simulink model "TST_WESDem_CalcState"  (R2016b)
settings: Solver=FixedStepDiscrete  StartTime=0.0  StopTime=simTime  FixedStep=sampleTime  RelTol=1e-3
values from neighbouring files (symbols this model uses):
  testCase = 1    [initTST_WESDem_CalcState_001.m]    (also in initTST_WESDem_CalcState_002.m = 2; initTST_WESDem_CalcState_003.m = 3)
libraries: simulink x25, UnitTest_Lib x21
(part 1 of 2)
settings Model: Creator=zhengjinyan  LastModifiedBy=zhengjinyan
settings DebuggingCC: SignalRangeChecking=error

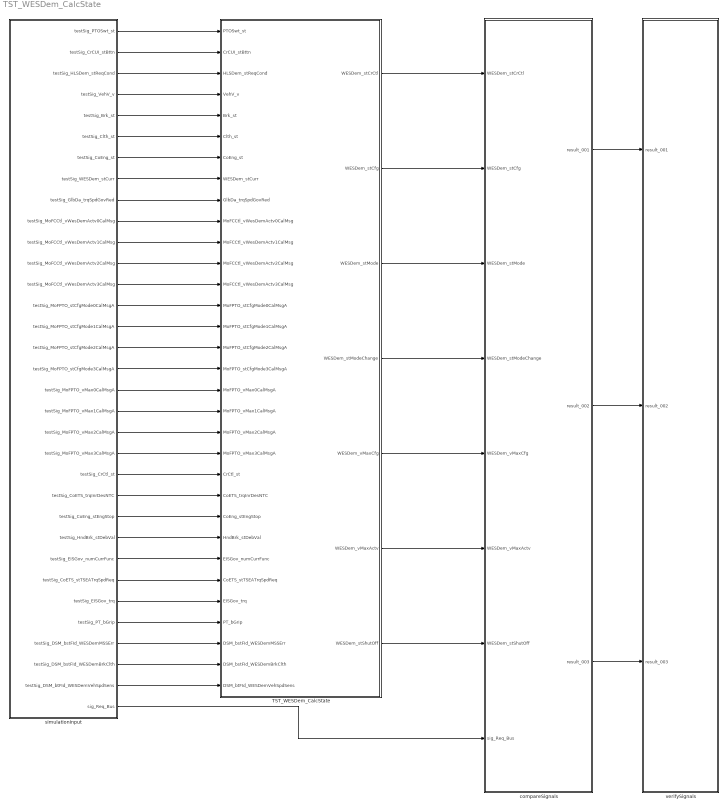
== system TST_WESDem_CalcState ==
  TST_WESDem_CalcState : Subsystem
  compareSignals : Subsystem
  simulationInput : Subsystem
  verifySignals : Subsystem
  wires:
  simulationInput/1(testSig_PTOSwt_st) -> TST_WESDem_CalcState/1(PTOSwt_st)
  simulationInput/2(testSig_CrCUI_stBttn) -> TST_WESDem_CalcState/2(CrCUI_stBttn)
  simulationInput/3(testSig_HLSDem_stReqCond) -> TST_WESDem_CalcState/3(HLSDem_stReqCond)
  simulationInput/4(testSig_VehV_v) -> TST_WESDem_CalcState/4(VehV_v)
  simulationInput/5(testSig_Brk_st) -> TST_WESDem_CalcState/5(Brk_st)
  simulationInput/6(testSig_Clth_st) -> TST_WESDem_CalcState/6(Clth_st)
  simulationInput/7(testSig_CoEng_st) -> TST_WESDem_CalcState/7(CoEng_st)
  simulationInput/8(testSig_WESDem_stCurr) -> TST_WESDem_CalcState/8(WESDem_stCurr)
  simulationInput/9(testSig_GlbDa_trqSpdGovRed) -> TST_WESDem_CalcState/9(GlbDa_trqSpdGovRed)
  simulationInput/10(testSig_MoFCCtl_vWesDemActv0CalMsg) -> TST_WESDem_CalcState/10(MoFCCtl_vWesDemActv0CalMsg)
  simulationInput/11(testSig_MoFCCtl_vWesDemActv1CalMsg) -> TST_WESDem_CalcState/11(MoFCCtl_vWesDemActv1CalMsg)
  simulationInput/12(testSig_MoFCCtl_vWesDemActv2CalMsg) -> TST_WESDem_CalcState/12(MoFCCtl_vWesDemActv2CalMsg)
  simulationInput/13(testSig_MoFCCtl_vWesDemActv3CalMsg) -> TST_WESDem_CalcState/13(MoFCCtl_vWesDemActv3CalMsg)
  simulationInput/14(testSig_MoFPTO_stCfgMode0CalMsgA) -> TST_WESDem_CalcState/14(MoFPTO_stCfgMode0CalMsgA)
  simulationInput/15(testSig_MoFPTO_stCfgMode1CalMsgA) -> TST_WESDem_CalcState/15(MoFPTO_stCfgMode1CalMsgA)
  simulationInput/16(testSig_MoFPTO_stCfgMode2CalMsgA) -> TST_WESDem_CalcState/16(MoFPTO_stCfgMode2CalMsgA)
  simulationInput/17(testSig_MoFPTO_stCfgMode3CalMsgA) -> TST_WESDem_CalcState/17(MoFPTO_stCfgMode3CalMsgA)
  simulationInput/18(testSig_MoFPTO_vMax0CalMsgA) -> TST_WESDem_CalcState/18(MoFPTO_vMax0CalMsgA)
  simulationInput/19(testSig_MoFPTO_vMax1CalMsgA) -> TST_WESDem_CalcState/19(MoFPTO_vMax1CalMsgA)
  simulationInput/20(testSig_MoFPTO_vMax2CalMsgA) -> TST_WESDem_CalcState/20(MoFPTO_vMax2CalMsgA)
  simulationInput/21(testSig_MoFPTO_vMax3CalMsgA) -> TST_WESDem_CalcState/21(MoFPTO_vMax3CalMsgA)
  simulationInput/22(testSig_CrCtl_st) -> TST_WESDem_CalcState/22(CrCtl_st)
  simulationInput/23(testSig_CoETS_trqInrDesNTC) -> TST_WESDem_CalcState/23(CoETS_trqInrDesNTC)
  simulationInput/24(testSig_CoEng_stEngStop) -> TST_WESDem_CalcState/24(CoEng_stEngStop)
  simulationInput/25(testSig_HndBrk_stDebVal) -> TST_WESDem_CalcState/25(HndBrk_stDebVal)
  simulationInput/26(testSig_EISGov_numCurrFunc) -> TST_WESDem_CalcState/26(EISGov_numCurrFunc)
  simulationInput/27(testSig_CoETS_stTSEATrqSpdReq) -> TST_WESDem_CalcState/27(CoETS_stTSEATrqSpdReq)
  simulationInput/28(testSig_EISGov_trq) -> TST_WESDem_CalcState/28(EISGov_trq)
  simulationInput/29(testSig_PT_bGrip) -> TST_WESDem_CalcState/29(PT_bGrip)
  simulationInput/30(testSig_DSM_bstFId_WESDemMSSErr) -> TST_WESDem_CalcState/30(DSM_bstFId_WESDemMSSErr)
  simulationInput/31(testSig_DSM_bstFId_WESDemBrkClth) -> TST_WESDem_CalcState/31(DSM_bstFId_WESDemBrkClth)
  simulationInput/32(testSig_DSM_btFId_WESDemVehSpdSens) -> TST_WESDem_CalcState/32(DSM_btFId_WESDemVehSpdSens)
  TST_WESDem_CalcState/1(WESDem_stCrCtl) -> compareSignals/1(WESDem_stCrCtl)
  TST_WESDem_CalcState/2(WESDem_stCfg) -> compareSignals/2(WESDem_stCfg)
  TST_WESDem_CalcState/3(WESDem_stMode) -> compareSignals/3(WESDem_stMode)
  TST_WESDem_CalcState/4(WESDem_stModeChange) -> compareSignals/4(WESDem_stModeChange)
  TST_WESDem_CalcState/5(WESDem_vMaxCfg) -> compareSignals/5(WESDem_vMaxCfg)
  TST_WESDem_CalcState/6(WESDem_vMaxActv) -> compareSignals/6(WESDem_vMaxActv)
  TST_WESDem_CalcState/7(WESDem_stShutOff) -> compareSignals/7(WESDem_stShutOff)
  simulationInput/33(sig_Req_Bus) -> compareSignals/8(sig_Req_Bus)
  compareSignals/1(result_001) -> verifySignals/1(result_001)
  compareSignals/2(result_002) -> verifySignals/2(result_002)
  compareSignals/3(result_003) -> verifySignals/3(result_003)

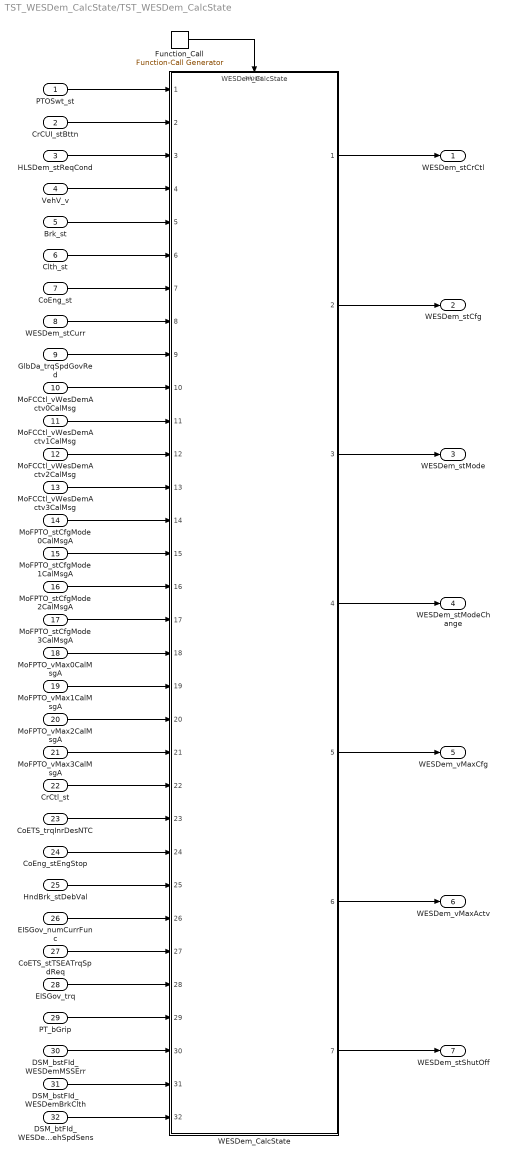
== system TST_WESDem_CalcState/TST_WESDem_CalcState ==
  PTOSwt_st : Inport
  CrCUI_stBttn : Inport  Port=2
  HLSDem_stReqCond : Inport  Port=3
  VehV_v : Inport  Port=4
  Brk_st : Inport  Port=5
  Clth_st : Inport  Port=6
  CoEng_st : Inport  Port=7
  WESDem_stCurr : Inport  Port=8
  GlbDa_trqSpdGovRed : Inport  Port=9
  MoFCCtl_vWesDemActv0CalMsg : Inport  Port=10
  MoFCCtl_vWesDemActv1CalMsg : Inport  Port=11
  MoFCCtl_vWesDemActv2CalMsg : Inport  Port=12
  MoFCCtl_vWesDemActv3CalMsg : Inport  Port=13
  MoFPTO_stCfgMode0CalMsgA : Inport  Port=14
  MoFPTO_stCfgMode1CalMsgA : Inport  Port=15
  MoFPTO_stCfgMode2CalMsgA : Inport  Port=16
  MoFPTO_stCfgMode3CalMsgA : Inport  Port=17
  MoFPTO_vMax0CalMsgA : Inport  Port=18
  MoFPTO_vMax1CalMsgA : Inport  Port=19
  MoFPTO_vMax2CalMsgA : Inport  Port=20
  MoFPTO_vMax3CalMsgA : Inport  Port=21
  CrCtl_st : Inport  Port=22
  CoETS_trqInrDesNTC : Inport  Port=23
  CoEng_stEngStop : Inport  Port=24
  HndBrk_stDebVal : Inport  Port=25
  EISGov_numCurrFunc : Inport  Port=26
  CoETS_stTSEATrqSpdReq : Inport  Port=27
  EISGov_trq : Inport  Port=28
  PT_bGrip : Inport  Port=29
  DSM_bstFId_WESDemMSSErr : Inport  Port=30
  DSM_bstFId_WESDemBrkClth : Inport  Port=31
  DSM_btFId_WESDemVehSpdSens : Inport  Port=32
  Function_Call : simulink/Ports & Subsystems/Function-Call Generator  sample_time=sampleTime  numberOfIterations=1
  WESDem_CalcState : ModelReference  ModelNameDialog=WESDem_CalcState  SimulationMode=Normal  ModelReferenceVersion=1.157  TriggerPortName=function  TriggerPortTriggerType=function-call  TriggerPortStatesWhenEnabling=held
  WESDem_stCrCtl : Outport
  WESDem_stCfg : Outport  Port=2
  WESDem_stMode : Outport  Port=3
  WESDem_stModeChange : Outport  Port=4
  WESDem_vMaxCfg : Outport  Port=5
  WESDem_vMaxActv : Outport  Port=6
  WESDem_stShutOff : Outport  Port=7
  wires:
  Function_Call/1 -> WESDem_CalcState/Trigger
  PTOSwt_st/1 -> WESDem_CalcState/1
  CrCUI_stBttn/1 -> WESDem_CalcState/2
  HLSDem_stReqCond/1 -> WESDem_CalcState/3
  VehV_v/1 -> WESDem_CalcState/4
  Brk_st/1 -> WESDem_CalcState/5
  Clth_st/1 -> WESDem_CalcState/6
  CoEng_st/1 -> WESDem_CalcState/7
  WESDem_stCurr/1 -> WESDem_CalcState/8
  GlbDa_trqSpdGovRed/1 -> WESDem_CalcState/9
  MoFCCtl_vWesDemActv0CalMsg/1 -> WESDem_CalcState/10
  MoFCCtl_vWesDemActv1CalMsg/1 -> WESDem_CalcState/11
  MoFCCtl_vWesDemActv2CalMsg/1 -> WESDem_CalcState/12
  MoFCCtl_vWesDemActv3CalMsg/1 -> WESDem_CalcState/13
  MoFPTO_stCfgMode0CalMsgA/1 -> WESDem_CalcState/14
  MoFPTO_stCfgMode1CalMsgA/1 -> WESDem_CalcState/15
  MoFPTO_stCfgMode2CalMsgA/1 -> WESDem_CalcState/16
  MoFPTO_stCfgMode3CalMsgA/1 -> WESDem_CalcState/17
  MoFPTO_vMax0CalMsgA/1 -> WESDem_CalcState/18
  MoFPTO_vMax1CalMsgA/1 -> WESDem_CalcState/19
  MoFPTO_vMax2CalMsgA/1 -> WESDem_CalcState/20
  MoFPTO_vMax3CalMsgA/1 -> WESDem_CalcState/21
  CrCtl_st/1 -> WESDem_CalcState/22
  CoETS_trqInrDesNTC/1 -> WESDem_CalcState/23
  CoEng_stEngStop/1 -> WESDem_CalcState/24
  HndBrk_stDebVal/1 -> WESDem_CalcState/25
  EISGov_numCurrFunc/1 -> WESDem_CalcState/26
  CoETS_stTSEATrqSpdReq/1 -> WESDem_CalcState/27
  EISGov_trq/1 -> WESDem_CalcState/28
  PT_bGrip/1 -> WESDem_CalcState/29
  DSM_bstFId_WESDemMSSErr/1 -> WESDem_CalcState/30
  DSM_bstFId_WESDemBrkClth/1 -> WESDem_CalcState/31
  DSM_btFId_WESDemVehSpdSens/1 -> WESDem_CalcState/32
  WESDem_CalcState/1 -> WESDem_stCrCtl/1
  WESDem_CalcState/2 -> WESDem_stCfg/1
  WESDem_CalcState/3 -> WESDem_stMode/1
  WESDem_CalcState/4 -> WESDem_stModeChange/1
  WESDem_CalcState/5 -> WESDem_vMaxCfg/1
  WESDem_CalcState/6 -> WESDem_vMaxActv/1
  WESDem_CalcState/7 -> WESDem_stShutOff/1

== system TST_WESDem_CalcState/compareSignals ==
  WESDem_stCrCtl : Inport
  WESDem_stCfg : Inport  Port=2
  WESDem_stMode : Inport  Port=3
  WESDem_stModeChange : Inport  Port=4
  WESDem_vMaxCfg : Inport  Port=5
  WESDem_vMaxActv : Inport  Port=6
  WESDem_stShutOff : Inport  Port=7
  sig_Req_Bus : Inport  Port=8
  BC : BusCreator  Inputs=7
  CTC_001 : simulink/Logic and Bit Operations/Compare To Constant  relop===  const=1  OutDataTypeStr=boolean
  CTC_002 : simulink/Logic and Bit Operations/Compare To Constant  relop===  const=2  OutDataTypeStr=boolean
  CTC_003 : simulink/Logic and Bit Operations/Compare To Constant  relop===  const=3  OutDataTypeStr=boolean
  Requirement_001 : Subsystem
  Requirement_002 : Subsystem
  Requirement_003 : Subsystem
  TC_001 : Constant  Value=testCase
  TC_002 : Constant  Value=testCase
  TC_003 : Constant  Value=testCase
  result_001 : Outport
  result_002 : Outport  Port=2
  result_003 : Outport  Port=3
  wires:
  WESDem_stCrCtl/1 -> BC/1  "WESDem_stCrCtl"
  WESDem_stCfg/1 -> BC/2  "WESDem_stCfg"
  WESDem_stMode/1 -> BC/3  "WESDem_stMode"
  WESDem_stModeChange/1 -> BC/4  "WESDem_stModeChange"
  WESDem_vMaxCfg/1 -> BC/5  "WESDem_vMaxCfg"
  WESDem_vMaxActv/1 -> BC/6  "WESDem_vMaxActv"
  WESDem_stShutOff/1 -> BC/7  "WESDem_stShutOff"
  TC_001/1 -> CTC_001/1
  CTC_001/1 -> Requirement_001/Enable
  sig_Req_Bus/1 -> Requirement_001/2(sig_Req_Bus), Requirement_002/2(sig_Req_Bus), Requirement_003/2(sig_Req_Bus)
  BC/1 -> Requirement_001/1(sig_Result_Bus), Requirement_002/1(sig_Result_Bus), Requirement_003/1(sig_Result_Bus)
  Requirement_001/1(result) -> result_001/1
  TC_002/1 -> CTC_002/1
  CTC_002/1 -> Requirement_002/Enable
  Requirement_002/1(result) -> result_002/1
  TC_003/1 -> CTC_003/1
  CTC_003/1 -> Requirement_003/Enable
  Requirement_003/1(result) -> result_003/1

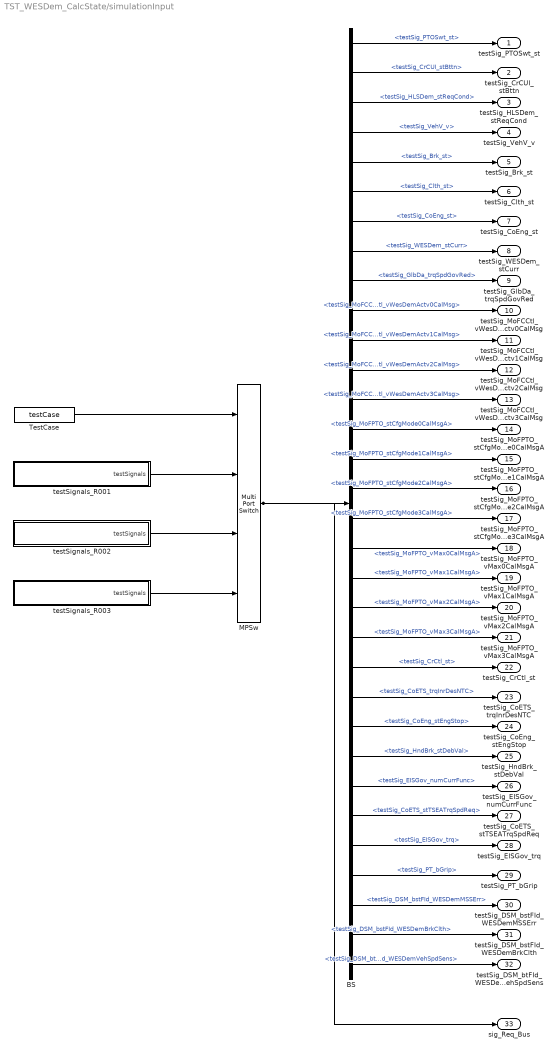
== system TST_WESDem_CalcState/simulationInput ==
  BS : BusSelector  OutputSignals=testSig_PTOSwt_st,testSig_CrCUI_stBttn,testSig_HLSDem_stReqCond,testSig_VehV_v,testSig_Brk_st,testSig_Clth_st,testSig_CoEng_st,testSig_WESDem_stCurr,testSig_GlbDa_trqSpdGovRed,testSig_MoFCCtl_vWesDemActv0CalMsg,testSig_MoFCCtl_vWesDemActv1CalMsg,testSig_MoFCCtl_vWesDemActv2CalMsg,testSig_MoFCCtl_vWesDemActv3CalMsg,testSig_MoFPTO_stCfgMode0CalMsgA,testSig_MoFPTO_stCfgMode1CalMsgA,testSig_MoFPTO_stCfgMode2CalMsgA,testSig_MoFPTO_stCfgMode3CalMsgA,testSig_MoFPTO_vMax0CalMsgA,testSig_MoFPTO_vMax1CalMsgA,testSig_MoFPTO_vMax2CalMsgA,testSig_MoFPTO_vMax3CalMsgA,testSig_CrCtl_st,testSig_CoETS_trqInrDesNTC,testSig_CoEng_stEngStop,testSig_HndBrk_stDebVal,testSig_EISGov_numCurrFunc,testSig_CoETS_stTSEATrqSpdReq,testSig_EISGov_trq,testSig_PT_bGrip,testSig_DSM_bstFId_WESDemMSSErr,testSig_DSM_bstFId_WESDemBrkClth,testSig_DSM_btFId_WESDemVehSpdSens
  MPSw : MultiPortSwitch  SaturateOnIntegerOverflow=on  InputSameDT=on
  TestCase : Constant  Value=testCase
  testSignals_R001 : Subsystem
  testSignals_R002 : Subsystem
  testSignals_R003 : Subsystem
  testSig_PTOSwt_st : Outport
  testSig_CrCUI_stBttn : Outport  Port=2
  testSig_HLSDem_stReqCond : Outport  Port=3
  testSig_VehV_v : Outport  Port=4
  testSig_Brk_st : Outport  Port=5
  testSig_Clth_st : Outport  Port=6
  testSig_CoEng_st : Outport  Port=7
  testSig_WESDem_stCurr : Outport  Port=8
  testSig_GlbDa_trqSpdGovRed : Outport  Port=9
  testSig_MoFCCtl_vWesDemActv0CalMsg : Outport  Port=10
  testSig_MoFCCtl_vWesDemActv1CalMsg : Outport  Port=11
  testSig_MoFCCtl_vWesDemActv2CalMsg : Outport  Port=12
  testSig_MoFCCtl_vWesDemActv3CalMsg : Outport  Port=13
  testSig_MoFPTO_stCfgMode0CalMsgA : Outport  Port=14
  testSig_MoFPTO_stCfgMode1CalMsgA : Outport  Port=15
  testSig_MoFPTO_stCfgMode2CalMsgA : Outport  Port=16
  testSig_MoFPTO_stCfgMode3CalMsgA : Outport  Port=17
  testSig_MoFPTO_vMax0CalMsgA : Outport  Port=18
  testSig_MoFPTO_vMax1CalMsgA : Outport  Port=19
  testSig_MoFPTO_vMax2CalMsgA : Outport  Port=20
  testSig_MoFPTO_vMax3CalMsgA : Outport  Port=21
  testSig_CrCtl_st : Outport  Port=22
  testSig_CoETS_trqInrDesNTC : Outport  Port=23
  testSig_CoEng_stEngStop : Outport  Port=24
  testSig_HndBrk_stDebVal : Outport  Port=25
  testSig_EISGov_numCurrFunc : Outport  Port=26
  testSig_CoETS_stTSEATrqSpdReq : Outport  Port=27
  testSig_EISGov_trq : Outport  Port=28
  testSig_PT_bGrip : Outport  Port=29
  testSig_DSM_bstFId_WESDemMSSErr : Outport  Port=30
  testSig_DSM_bstFId_WESDemBrkClth : Outport  Port=31
  testSig_DSM_btFId_WESDemVehSpdSens : Outport  Port=32
  sig_Req_Bus : Outport  Port=33
  wires:
  BS/1 -> testSig_PTOSwt_st/1  "<testSig_PTOSwt_st>"
  BS/2 -> testSig_CrCUI_stBttn/1  "<testSig_CrCUI_stBttn>"
  BS/3 -> testSig_HLSDem_stReqCond/1  "<testSig_HLSDem_stReqCond>"
  BS/4 -> testSig_VehV_v/1  "<testSig_VehV_v>"
  BS/5 -> testSig_Brk_st/1  "<testSig_Brk_st>"
  BS/6 -> testSig_Clth_st/1  "<testSig_Clth_st>"
  BS/7 -> testSig_CoEng_st/1  "<testSig_CoEng_st>"
  BS/8 -> testSig_WESDem_stCurr/1  "<testSig_WESDem_stCurr>"
  BS/9 -> testSig_GlbDa_trqSpdGovRed/1  "<testSig_GlbDa_trqSpdGovRed>"
  BS/10 -> testSig_MoFCCtl_vWesDemActv0CalMsg/1  "<testSig_MoFCCtl_vWesDemActv0CalMsg>"
  BS/11 -> testSig_MoFCCtl_vWesDemActv1CalMsg/1  "<testSig_MoFCCtl_vWesDemActv1CalMsg>"
  BS/12 -> testSig_MoFCCtl_vWesDemActv2CalMsg/1  "<testSig_MoFCCtl_vWesDemActv2CalMsg>"
  BS/13 -> testSig_MoFCCtl_vWesDemActv3CalMsg/1  "<testSig_MoFCCtl_vWesDemActv3CalMsg>"
  BS/14 -> testSig_MoFPTO_stCfgMode0CalMsgA/1  "<testSig_MoFPTO_stCfgMode0CalMsgA>"
  BS/15 -> testSig_MoFPTO_stCfgMode1CalMsgA/1  "<testSig_MoFPTO_stCfgMode1CalMsgA>"
  BS/16 -> testSig_MoFPTO_stCfgMode2CalMsgA/1  "<testSig_MoFPTO_stCfgMode2CalMsgA>"
  BS/17 -> testSig_MoFPTO_stCfgMode3CalMsgA/1  "<testSig_MoFPTO_stCfgMode3CalMsgA>"
  BS/18 -> testSig_MoFPTO_vMax0CalMsgA/1  "<testSig_MoFPTO_vMax0CalMsgA>"
  BS/19 -> testSig_MoFPTO_vMax1CalMsgA/1  "<testSig_MoFPTO_vMax1CalMsgA>"
  BS/20 -> testSig_MoFPTO_vMax2CalMsgA/1  "<testSig_MoFPTO_vMax2CalMsgA>"
  BS/21 -> testSig_MoFPTO_vMax3CalMsgA/1  "<testSig_MoFPTO_vMax3CalMsgA>"
  BS/22 -> testSig_CrCtl_st/1  "<testSig_CrCtl_st>"
  BS/23 -> testSig_CoETS_trqInrDesNTC/1  "<testSig_CoETS_trqInrDesNTC>"
  BS/24 -> testSig_CoEng_stEngStop/1  "<testSig_CoEng_stEngStop>"
  BS/25 -> testSig_HndBrk_stDebVal/1  "<testSig_HndBrk_stDebVal>"
  BS/26 -> testSig_EISGov_numCurrFunc/1  "<testSig_EISGov_numCurrFunc>"
  BS/27 -> testSig_CoETS_stTSEATrqSpdReq/1  "<testSig_CoETS_stTSEATrqSpdReq>"
  BS/28 -> testSig_EISGov_trq/1  "<testSig_EISGov_trq>"
  BS/29 -> testSig_PT_bGrip/1  "<testSig_PT_bGrip>"
  BS/30 -> testSig_DSM_bstFId_WESDemMSSErr/1  "<testSig_DSM_bstFId_WESDemMSSErr>"
  BS/31 -> testSig_DSM_bstFId_WESDemBrkClth/1  "<testSig_DSM_bstFId_WESDemBrkClth>"
  BS/32 -> testSig_DSM_btFId_WESDemVehSpdSens/1  "<testSig_DSM_btFId_WESDemVehSpdSens>"
  MPSw/1 -> BS/1, sig_Req_Bus/1
  TestCase/1 -> MPSw/1
  testSignals_R001/1(testSignals) -> MPSw/2
  testSignals_R002/1(testSignals) -> MPSw/3
  testSignals_R003/1(testSignals) -> MPSw/4

== system TST_WESDem_CalcState/verifySignals ==
  result_001 : Inport
  result_002 : Inport  Port=2
  result_003 : Inport  Port=3
  Assertion_001 : Assertion  Enabled=off
  Assertion_002 : Assertion  Enabled=off
  Assertion_003 : Assertion  Enabled=off
  wires:
  result_001/1 -> Assertion_001/1
  result_002/1 -> Assertion_002/1
  result_003/1 -> Assertion_003/1

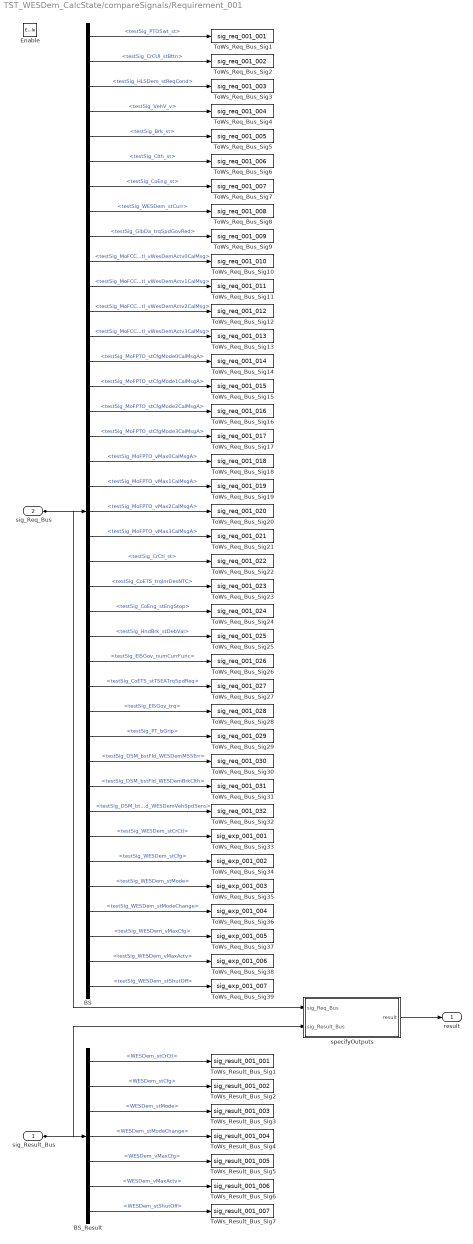
== system TST_WESDem_CalcState/compareSignals/Requirement_001 ==
  sig_Result_Bus : Inport
  sig_Req_Bus : Inport  Port=2
  Enable : EnablePort
  BS : BusSelector  OutputSignals=testSig_PTOSwt_st,testSig_CrCUI_stBttn,testSig_HLSDem_stReqCond,testSig_VehV_v,testSig_Brk_st,testSig_Clth_st,testSig_CoEng_st,testSig_WESDem_stCurr,testSig_GlbDa_trqSpdGovRed,testSig_MoFCCtl_vWesDemActv0CalMsg,testSig_MoFCCtl_vWesDemActv1CalMsg,testSig_MoFCCtl_vWesDemActv2CalMsg,testSig_MoFCCtl_vWesDemActv3CalMsg,testSig_MoFPTO_stCfgMode0CalMsgA,testSig_MoFPTO_stCfgMode1CalMsgA,testSig_MoFPTO_stCfgMode2CalMsgA,testSig_MoFPTO_stCfgMode3CalMsgA,testSig_MoFPTO_vMax0CalMsgA,testSig_MoFPTO_vMax1CalMsgA,testSig_MoFPTO_vMax2CalMsgA,testSig_MoFPTO_vMax3CalMsgA,testSig_CrCtl_st,testSig_CoETS_trqInrDesNTC,testSig_CoEng_stEngStop,testSig_HndBrk_stDebVal,testSig_EISGov_numCurrFunc,testSig_CoETS_stTSEATrqSpdReq,testSig_EISGov_trq,testSig_PT_bGrip,testSig_DSM_bstFId_WESDemMSSErr,testSig_DSM_bstFId_WESDemBrkClth,testSig_DSM_btFId_WESDemVehSpdSens,testSig_WESDem_stCrCtl,testSig_WESDem_stCfg,testSig_WESDem_stMode,testSig_WESDem_stModeChange,testSig_WESDem_vMaxCfg,testSig_WESDem_vMaxActv,testSig_WESDem_stShutOff
  BS_Result : BusSelector  OutputSignals=WESDem_stCrCtl,WESDem_stCfg,WESDem_stMode,WESDem_stModeChange,WESDem_vMaxCfg,WESDem_vMaxActv,WESDem_stShutOff
  ToWs_Req_Bus_Sig1 : ToWorkspace  VariableName=sig_req_001_001  SaveFormat=Structure With Time
  ToWs_Req_Bus_Sig10 : ToWorkspace  VariableName=sig_req_001_010  SaveFormat=Structure With Time
  ToWs_Req_Bus_Sig11 : ToWorkspace  VariableName=sig_req_001_011  SaveFormat=Structure With Time
  ToWs_Req_Bus_Sig12 : ToWorkspace  VariableName=sig_req_001_012  SaveFormat=Structure With Time
  ToWs_Req_Bus_Sig13 : ToWorkspace  VariableName=sig_req_001_013  SaveFormat=Structure With Time
  ToWs_Req_Bus_Sig14 : ToWorkspace  VariableName=sig_req_001_014  SaveFormat=Structure With Time
  ToWs_Req_Bus_Sig15 : ToWorkspace  VariableName=sig_req_001_015  SaveFormat=Structure With Time
  ToWs_Req_Bus_Sig16 : ToWorkspace  VariableName=sig_req_001_016  SaveFormat=Structure With Time
  ToWs_Req_Bus_Sig17 : ToWorkspace  VariableName=sig_req_001_017  SaveFormat=Structure With Time
  ToWs_Req_Bus_Sig18 : ToWorkspace  VariableName=sig_req_001_018  SaveFormat=Structure With Time
  ToWs_Req_Bus_Sig19 : ToWorkspace  VariableName=sig_req_001_019  SaveFormat=Structure With Time
  ToWs_Req_Bus_Sig2 : ToWorkspace  VariableName=sig_req_001_002  SaveFormat=Structure With Time
  ToWs_Req_Bus_Sig20 : ToWorkspace  VariableName=sig_req_001_020  SaveFormat=Structure With Time
  ToWs_Req_Bus_Sig21 : ToWorkspace  VariableName=sig_req_001_021  SaveFormat=Structure With Time
  ToWs_Req_Bus_Sig22 : ToWorkspace  VariableName=sig_req_001_022  SaveFormat=Structure With Time
  ToWs_Req_Bus_Sig23 : ToWorkspace  VariableName=sig_req_001_023  SaveFormat=Structure With Time
  ToWs_Req_Bus_Sig24 : ToWorkspace  VariableName=sig_req_001_024  SaveFormat=Structure With Time
  ToWs_Req_Bus_Sig25 : ToWorkspace  VariableName=sig_req_001_025  SaveFormat=Structure With Time
  ToWs_Req_Bus_Sig26 : ToWorkspace  VariableName=sig_req_001_026  SaveFormat=Structure With Time
  ToWs_Req_Bus_Sig27 : ToWorkspace  VariableName=sig_req_001_027  SaveFormat=Structure With Time
  ToWs_Req_Bus_Sig28 : ToWorkspace  VariableName=sig_req_001_028  SaveFormat=Structure With Time
  ToWs_Req_Bus_Sig29 : ToWorkspace  VariableName=sig_req_001_029  SaveFormat=Structure With Time
  ToWs_Req_Bus_Sig3 : ToWorkspace  VariableName=sig_req_001_003  SaveFormat=Structure With Time
  ToWs_Req_Bus_Sig30 : ToWorkspace  VariableName=sig_req_001_030  SaveFormat=Structure With Time
  ToWs_Req_Bus_Sig31 : ToWorkspace  VariableName=sig_req_001_031  SaveFormat=Structure With Time
  ToWs_Req_Bus_Sig32 : ToWorkspace  VariableName=sig_req_001_032  SaveFormat=Structure With Time
  ToWs_Req_Bus_Sig33 : ToWorkspace  VariableName=sig_exp_001_001  SaveFormat=Structure With Time
  ToWs_Req_Bus_Sig34 : ToWorkspace  VariableName=sig_exp_001_002  SaveFormat=Structure With Time
  ToWs_Req_Bus_Sig35 : ToWorkspace  VariableName=sig_exp_001_003  SaveFormat=Structure With Time
  ToWs_Req_Bus_Sig36 : ToWorkspace  VariableName=sig_exp_001_004  SaveFormat=Structure With Time
  ToWs_Req_Bus_Sig37 : ToWorkspace  VariableName=sig_exp_001_005  SaveFormat=Structure With Time
  ToWs_Req_Bus_Sig38 : ToWorkspace  VariableName=sig_exp_001_006  SaveFormat=Structure With Time
  ToWs_Req_Bus_Sig39 : ToWorkspace  VariableName=sig_exp_001_007  SaveFormat=Structure With Time
  ToWs_Req_Bus_Sig4 : ToWorkspace  VariableName=sig_req_001_004  SaveFormat=Structure With Time
  ToWs_Req_Bus_Sig5 : ToWorkspace  VariableName=sig_req_001_005  SaveFormat=Structure With Time
  ToWs_Req_Bus_Sig6 : ToWorkspace  VariableName=sig_req_001_006  SaveFormat=Structure With Time
  ToWs_Req_Bus_Sig7 : ToWorkspace  VariableName=sig_req_001_007  SaveFormat=Structure With Time
  ToWs_Req_Bus_Sig8 : ToWorkspace  VariableName=sig_req_001_008  SaveFormat=Structure With Time
  ToWs_Req_Bus_Sig9 : ToWorkspace  VariableName=sig_req_001_009  SaveFormat=Structure With Time
  ToWs_Result_Bus_Sig1 : ToWorkspace  VariableName=sig_result_001_001  SaveFormat=Structure With Time
  ToWs_Result_Bus_Sig2 : ToWorkspace  VariableName=sig_result_001_002  SaveFormat=Structure With Time
  ToWs_Result_Bus_Sig3 : ToWorkspace  VariableName=sig_result_001_003  SaveFormat=Structure With Time
  ToWs_Result_Bus_Sig4 : ToWorkspace  VariableName=sig_result_001_004  SaveFormat=Structure With Time
  ToWs_Result_Bus_Sig5 : ToWorkspace  VariableName=sig_result_001_005  SaveFormat=Structure With Time
  ToWs_Result_Bus_Sig6 : ToWorkspace  VariableName=sig_result_001_006  SaveFormat=Structure With Time
  ToWs_Result_Bus_Sig7 : ToWorkspace  VariableName=sig_result_001_007  SaveFormat=Structure With Time
  specifyOutputs : Subsystem
  result : Outport
  wires:
  sig_Req_Bus/1 -> BS/1, specifyOutputs/1(sig_Req_Bus)
  BS/1 -> ToWs_Req_Bus_Sig1/1  "<testSig_PTOSwt_st>"
  BS/2 -> ToWs_Req_Bus_Sig2/1  "<testSig_CrCUI_stBttn>"
  BS/3 -> ToWs_Req_Bus_Sig3/1  "<testSig_HLSDem_stReqCond>"
  BS/4 -> ToWs_Req_Bus_Sig4/1  "<testSig_VehV_v>"
  BS/5 -> ToWs_Req_Bus_Sig5/1  "<testSig_Brk_st>"
  BS/6 -> ToWs_Req_Bus_Sig6/1  "<testSig_Clth_st>"
  BS/7 -> ToWs_Req_Bus_Sig7/1  "<testSig_CoEng_st>"
  BS/8 -> ToWs_Req_Bus_Sig8/1  "<testSig_WESDem_stCurr>"
  BS/9 -> ToWs_Req_Bus_Sig9/1  "<testSig_GlbDa_trqSpdGovRed>"
  BS/10 -> ToWs_Req_Bus_Sig10/1  "<testSig_MoFCCtl_vWesDemActv0CalMsg>"
  BS/11 -> ToWs_Req_Bus_Sig11/1  "<testSig_MoFCCtl_vWesDemActv1CalMsg>"
  BS/12 -> ToWs_Req_Bus_Sig12/1  "<testSig_MoFCCtl_vWesDemActv2CalMsg>"
  BS/13 -> ToWs_Req_Bus_Sig13/1  "<testSig_MoFCCtl_vWesDemActv3CalMsg>"
  BS/14 -> ToWs_Req_Bus_Sig14/1  "<testSig_MoFPTO_stCfgMode0CalMsgA>"
  BS/15 -> ToWs_Req_Bus_Sig15/1  "<testSig_MoFPTO_stCfgMode1CalMsgA>"
  BS/16 -> ToWs_Req_Bus_Sig16/1  "<testSig_MoFPTO_stCfgMode2CalMsgA>"
  BS/17 -> ToWs_Req_Bus_Sig17/1  "<testSig_MoFPTO_stCfgMode3CalMsgA>"
  BS/18 -> ToWs_Req_Bus_Sig18/1  "<testSig_MoFPTO_vMax0CalMsgA>"
  BS/19 -> ToWs_Req_Bus_Sig19/1  "<testSig_MoFPTO_vMax1CalMsgA>"
  BS/20 -> ToWs_Req_Bus_Sig20/1  "<testSig_MoFPTO_vMax2CalMsgA>"
  BS/21 -> ToWs_Req_Bus_Sig21/1  "<testSig_MoFPTO_vMax3CalMsgA>"
  BS/22 -> ToWs_Req_Bus_Sig22/1  "<testSig_CrCtl_st>"
  BS/23 -> ToWs_Req_Bus_Sig23/1  "<testSig_CoETS_trqInrDesNTC>"
  BS/24 -> ToWs_Req_Bus_Sig24/1  "<testSig_CoEng_stEngStop>"
  BS/25 -> ToWs_Req_Bus_Sig25/1  "<testSig_HndBrk_stDebVal>"
  BS/26 -> ToWs_Req_Bus_Sig26/1  "<testSig_EISGov_numCurrFunc>"
  BS/27 -> ToWs_Req_Bus_Sig27/1  "<testSig_CoETS_stTSEATrqSpdReq>"
  BS/28 -> ToWs_Req_Bus_Sig28/1  "<testSig_EISGov_trq>"
  BS/29 -> ToWs_Req_Bus_Sig29/1  "<testSig_PT_bGrip>"
  BS/30 -> ToWs_Req_Bus_Sig30/1  "<testSig_DSM_bstFId_WESDemMSSErr>"
  BS/31 -> ToWs_Req_Bus_Sig31/1  "<testSig_DSM_bstFId_WESDemBrkClth>"
  BS/32 -> ToWs_Req_Bus_Sig32/1  "<testSig_DSM_btFId_WESDemVehSpdSens>"
  BS/33 -> ToWs_Req_Bus_Sig33/1  "<testSig_WESDem_stCrCtl>"
  BS/34 -> ToWs_Req_Bus_Sig34/1  "<testSig_WESDem_stCfg>"
  BS/35 -> ToWs_Req_Bus_Sig35/1  "<testSig_WESDem_stMode>"
  BS/36 -> ToWs_Req_Bus_Sig36/1  "<testSig_WESDem_stModeChange>"
  BS/37 -> ToWs_Req_Bus_Sig37/1  "<testSig_WESDem_vMaxCfg>"
  BS/38 -> ToWs_Req_Bus_Sig38/1  "<testSig_WESDem_vMaxActv>"
  BS/39 -> ToWs_Req_Bus_Sig39/1  "<testSig_WESDem_stShutOff>"
  sig_Result_Bus/1 -> BS_Result/1, specifyOutputs/2(sig_Result_Bus)
  BS_Result/1 -> ToWs_Result_Bus_Sig1/1  "<WESDem_stCrCtl>"
  BS_Result/2 -> ToWs_Result_Bus_Sig2/1  "<WESDem_stCfg>"
  BS_Result/3 -> ToWs_Result_Bus_Sig3/1  "<WESDem_stMode>"
  BS_Result/4 -> ToWs_Result_Bus_Sig4/1  "<WESDem_stModeChange>"
  BS_Result/5 -> ToWs_Result_Bus_Sig5/1  "<WESDem_vMaxCfg>"
  BS_Result/6 -> ToWs_Result_Bus_Sig6/1  "<WESDem_vMaxActv>"
  BS_Result/7 -> ToWs_Result_Bus_Sig7/1  "<WESDem_stShutOff>"
  specifyOutputs/1(result) -> result/1

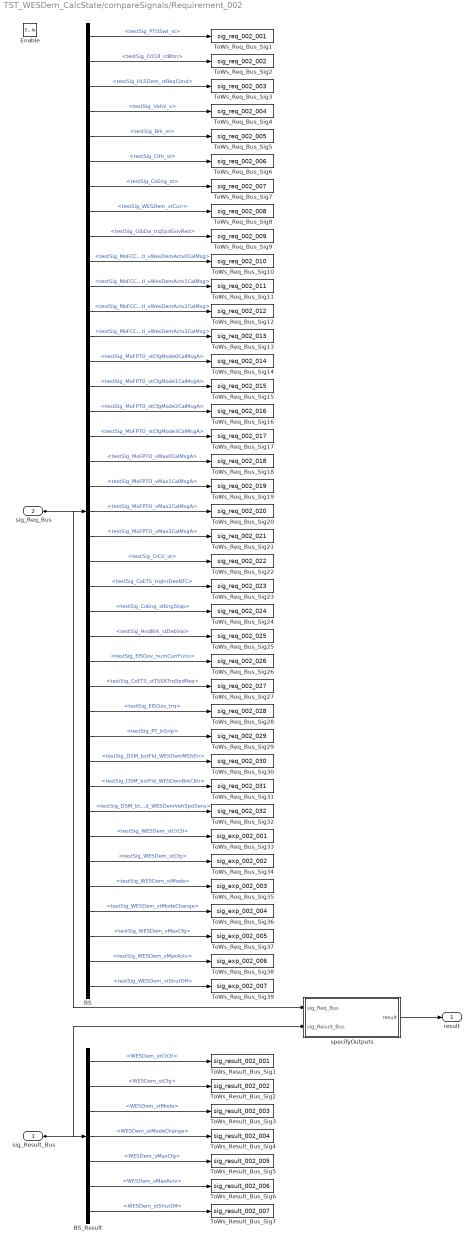
== system TST_WESDem_CalcState/compareSignals/Requirement_002 ==
  sig_Result_Bus : Inport
  sig_Req_Bus : Inport  Port=2
  Enable : EnablePort
  BS : BusSelector  OutputSignals=testSig_PTOSwt_st,testSig_CrCUI_stBttn,testSig_HLSDem_stReqCond,testSig_VehV_v,testSig_Brk_st,testSig_Clth_st,testSig_CoEng_st,testSig_WESDem_stCurr,testSig_GlbDa_trqSpdGovRed,testSig_MoFCCtl_vWesDemActv0CalMsg,testSig_MoFCCtl_vWesDemActv1CalMsg,testSig_MoFCCtl_vWesDemActv2CalMsg,testSig_MoFCCtl_vWesDemActv3CalMsg,testSig_MoFPTO_stCfgMode0CalMsgA,testSig_MoFPTO_stCfgMode1CalMsgA,testSig_MoFPTO_stCfgMode2CalMsgA,testSig_MoFPTO_stCfgMode3CalMsgA,testSig_MoFPTO_vMax0CalMsgA,testSig_MoFPTO_vMax1CalMsgA,testSig_MoFPTO_vMax2CalMsgA,testSig_MoFPTO_vMax3CalMsgA,testSig_CrCtl_st,testSig_CoETS_trqInrDesNTC,testSig_CoEng_stEngStop,testSig_HndBrk_stDebVal,testSig_EISGov_numCurrFunc,testSig_CoETS_stTSEATrqSpdReq,testSig_EISGov_trq,testSig_PT_bGrip,testSig_DSM_bstFId_WESDemMSSErr,testSig_DSM_bstFId_WESDemBrkClth,testSig_DSM_btFId_WESDemVehSpdSens,testSig_WESDem_stCrCtl,testSig_WESDem_stCfg,testSig_WESDem_stMode,testSig_WESDem_stModeChange,testSig_WESDem_vMaxCfg,testSig_WESDem_vMaxActv,testSig_WESDem_stShutOff
  BS_Result : BusSelector  OutputSignals=WESDem_stCrCtl,WESDem_stCfg,WESDem_stMode,WESDem_stModeChange,WESDem_vMaxCfg,WESDem_vMaxActv,WESDem_stShutOff
  ToWs_Req_Bus_Sig1 : ToWorkspace  VariableName=sig_req_002_001  SaveFormat=Structure With Time
  ToWs_Req_Bus_Sig10 : ToWorkspace  VariableName=sig_req_002_010  SaveFormat=Structure With Time
  ToWs_Req_Bus_Sig11 : ToWorkspace  VariableName=sig_req_002_011  SaveFormat=Structure With Time
  ToWs_Req_Bus_Sig12 : ToWorkspace  VariableName=sig_req_002_012  SaveFormat=Structure With Time
  ToWs_Req_Bus_Sig13 : ToWorkspace  VariableName=sig_req_002_013  SaveFormat=Structure With Time
  ToWs_Req_Bus_Sig14 : ToWorkspace  VariableName=sig_req_002_014  SaveFormat=Structure With Time
  ToWs_Req_Bus_Sig15 : ToWorkspace  VariableName=sig_req_002_015  SaveFormat=Structure With Time
  ToWs_Req_Bus_Sig16 : ToWorkspace  VariableName=sig_req_002_016  SaveFormat=Structure With Time
  ToWs_Req_Bus_Sig17 : ToWorkspace  VariableName=sig_req_002_017  SaveFormat=Structure With Time
  ToWs_Req_Bus_Sig18 : ToWorkspace  VariableName=sig_req_002_018  SaveFormat=Structure With Time
  ToWs_Req_Bus_Sig19 : ToWorkspace  VariableName=sig_req_002_019  SaveFormat=Structure With Time
  ToWs_Req_Bus_Sig2 : ToWorkspace  VariableName=sig_req_002_002  SaveFormat=Structure With Time
  ToWs_Req_Bus_Sig20 : ToWorkspace  VariableName=sig_req_002_020  SaveFormat=Structure With Time
  ToWs_Req_Bus_Sig21 : ToWorkspace  VariableName=sig_req_002_021  SaveFormat=Structure With Time
  ToWs_Req_Bus_Sig22 : ToWorkspace  VariableName=sig_req_002_022  SaveFormat=Structure With Time
  ToWs_Req_Bus_Sig23 : ToWorkspace  VariableName=sig_req_002_023  SaveFormat=Structure With Time
  ToWs_Req_Bus_Sig24 : ToWorkspace  VariableName=sig_req_002_024  SaveFormat=Structure With Time
  ToWs_Req_Bus_Sig25 : ToWorkspace  VariableName=sig_req_002_025  SaveFormat=Structure With Time
  ToWs_Req_Bus_Sig26 : ToWorkspace  VariableName=sig_req_002_026  SaveFormat=Structure With Time
  ToWs_Req_Bus_Sig27 : ToWorkspace  VariableName=sig_req_002_027  SaveFormat=Structure With Time
  ToWs_Req_Bus_Sig28 : ToWorkspace  VariableName=sig_req_002_028  SaveFormat=Structure With Time
  ToWs_Req_Bus_Sig29 : ToWorkspace  VariableName=sig_req_002_029  SaveFormat=Structure With Time
  ToWs_Req_Bus_Sig3 : ToWorkspace  VariableName=sig_req_002_003  SaveFormat=Structure With Time
  ToWs_Req_Bus_Sig30 : ToWorkspace  VariableName=sig_req_002_030  SaveFormat=Structure With Time
  ToWs_Req_Bus_Sig31 : ToWorkspace  VariableName=sig_req_002_031  SaveFormat=Structure With Time
  ToWs_Req_Bus_Sig32 : ToWorkspace  VariableName=sig_req_002_032  SaveFormat=Structure With Time
  ToWs_Req_Bus_Sig33 : ToWorkspace  VariableName=sig_exp_002_001  SaveFormat=Structure With Time
  ToWs_Req_Bus_Sig34 : ToWorkspace  VariableName=sig_exp_002_002  SaveFormat=Structure With Time
  ToWs_Req_Bus_Sig35 : ToWorkspace  VariableName=sig_exp_002_003  SaveFormat=Structure With Time
  ToWs_Req_Bus_Sig36 : ToWorkspace  VariableName=sig_exp_002_004  SaveFormat=Structure With Time
  ToWs_Req_Bus_Sig37 : ToWorkspace  VariableName=sig_exp_002_005  SaveFormat=Structure With Time
  ToWs_Req_Bus_Sig38 : ToWorkspace  VariableName=sig_exp_002_006  SaveFormat=Structure With Time
  ToWs_Req_Bus_Sig39 : ToWorkspace  VariableName=sig_exp_002_007  SaveFormat=Structure With Time
  ToWs_Req_Bus_Sig4 : ToWorkspace  VariableName=sig_req_002_004  SaveFormat=Structure With Time
  ToWs_Req_Bus_Sig5 : ToWorkspace  VariableName=sig_req_002_005  SaveFormat=Structure With Time
  ToWs_Req_Bus_Sig6 : ToWorkspace  VariableName=sig_req_002_006  SaveFormat=Structure With Time
  ToWs_Req_Bus_Sig7 : ToWorkspace  VariableName=sig_req_002_007  SaveFormat=Structure With Time
  ToWs_Req_Bus_Sig8 : ToWorkspace  VariableName=sig_req_002_008  SaveFormat=Structure With Time
  ToWs_Req_Bus_Sig9 : ToWorkspace  VariableName=sig_req_002_009  SaveFormat=Structure With Time
  ToWs_Result_Bus_Sig1 : ToWorkspace  VariableName=sig_result_002_001  SaveFormat=Structure With Time
  ToWs_Result_Bus_Sig2 : ToWorkspace  VariableName=sig_result_002_002  SaveFormat=Structure With Time
  ToWs_Result_Bus_Sig3 : ToWorkspace  VariableName=sig_result_002_003  SaveFormat=Structure With Time
  ToWs_Result_Bus_Sig4 : ToWorkspace  VariableName=sig_result_002_004  SaveFormat=Structure With Time
  ToWs_Result_Bus_Sig5 : ToWorkspace  VariableName=sig_result_002_005  SaveFormat=Structure With Time
  ToWs_Result_Bus_Sig6 : ToWorkspace  VariableName=sig_result_002_006  SaveFormat=Structure With Time
  ToWs_Result_Bus_Sig7 : ToWorkspace  VariableName=sig_result_002_007  SaveFormat=Structure With Time
  specifyOutputs : Subsystem
  result : Outport
  wires:
  sig_Req_Bus/1 -> BS/1, specifyOutputs/1(sig_Req_Bus)
  BS/1 -> ToWs_Req_Bus_Sig1/1  "<testSig_PTOSwt_st>"
  BS/2 -> ToWs_Req_Bus_Sig2/1  "<testSig_CrCUI_stBttn>"
  BS/3 -> ToWs_Req_Bus_Sig3/1  "<testSig_HLSDem_stReqCond>"
  BS/4 -> ToWs_Req_Bus_Sig4/1  "<testSig_VehV_v>"
  BS/5 -> ToWs_Req_Bus_Sig5/1  "<testSig_Brk_st>"
  BS/6 -> ToWs_Req_Bus_Sig6/1  "<testSig_Clth_st>"
  BS/7 -> ToWs_Req_Bus_Sig7/1  "<testSig_CoEng_st>"
  BS/8 -> ToWs_Req_Bus_Sig8/1  "<testSig_WESDem_stCurr>"
  BS/9 -> ToWs_Req_Bus_Sig9/1  "<testSig_GlbDa_trqSpdGovRed>"
  BS/10 -> ToWs_Req_Bus_Sig10/1  "<testSig_MoFCCtl_vWesDemActv0CalMsg>"
  BS/11 -> ToWs_Req_Bus_Sig11/1  "<testSig_MoFCCtl_vWesDemActv1CalMsg>"
  BS/12 -> ToWs_Req_Bus_Sig12/1  "<testSig_MoFCCtl_vWesDemActv2CalMsg>"
  BS/13 -> ToWs_Req_Bus_Sig13/1  "<testSig_MoFCCtl_vWesDemActv3CalMsg>"
  BS/14 -> ToWs_Req_Bus_Sig14/1  "<testSig_MoFPTO_stCfgMode0CalMsgA>"
  BS/15 -> ToWs_Req_Bus_Sig15/1  "<testSig_MoFPTO_stCfgMode1CalMsgA>"
  BS/16 -> ToWs_Req_Bus_Sig16/1  "<testSig_MoFPTO_stCfgMode2CalMsgA>"
  BS/17 -> ToWs_Req_Bus_Sig17/1  "<testSig_MoFPTO_stCfgMode3CalMsgA>"
  BS/18 -> ToWs_Req_Bus_Sig18/1  "<testSig_MoFPTO_vMax0CalMsgA>"
  BS/19 -> ToWs_Req_Bus_Sig19/1  "<testSig_MoFPTO_vMax1CalMsgA>"
  BS/20 -> ToWs_Req_Bus_Sig20/1  "<testSig_MoFPTO_vMax2CalMsgA>"
  BS/21 -> ToWs_Req_Bus_Sig21/1  "<testSig_MoFPTO_vMax3CalMsgA>"
  BS/22 -> ToWs_Req_Bus_Sig22/1  "<testSig_CrCtl_st>"
  BS/23 -> ToWs_Req_Bus_Sig23/1  "<testSig_CoETS_trqInrDesNTC>"
  BS/24 -> ToWs_Req_Bus_Sig24/1  "<testSig_CoEng_stEngStop>"
  BS/25 -> ToWs_Req_Bus_Sig25/1  "<testSig_HndBrk_stDebVal>"
  BS/26 -> ToWs_Req_Bus_Sig26/1  "<testSig_EISGov_numCurrFunc>"
  BS/27 -> ToWs_Req_Bus_Sig27/1  "<testSig_CoETS_stTSEATrqSpdReq>"
  BS/28 -> ToWs_Req_Bus_Sig28/1  "<testSig_EISGov_trq>"
  BS/29 -> ToWs_Req_Bus_Sig29/1  "<testSig_PT_bGrip>"
  BS/30 -> ToWs_Req_Bus_Sig30/1  "<testSig_DSM_bstFId_WESDemMSSErr>"
  BS/31 -> ToWs_Req_Bus_Sig31/1  "<testSig_DSM_bstFId_WESDemBrkClth>"
  BS/32 -> ToWs_Req_Bus_Sig32/1  "<testSig_DSM_btFId_WESDemVehSpdSens>"
  BS/33 -> ToWs_Req_Bus_Sig33/1  "<testSig_WESDem_stCrCtl>"
  BS/34 -> ToWs_Req_Bus_Sig34/1  "<testSig_WESDem_stCfg>"
  BS/35 -> ToWs_Req_Bus_Sig35/1  "<testSig_WESDem_stMode>"
  BS/36 -> ToWs_Req_Bus_Sig36/1  "<testSig_WESDem_stModeChange>"
  BS/37 -> ToWs_Req_Bus_Sig37/1  "<testSig_WESDem_vMaxCfg>"
  BS/38 -> ToWs_Req_Bus_Sig38/1  "<testSig_WESDem_vMaxActv>"
  BS/39 -> ToWs_Req_Bus_Sig39/1  "<testSig_WESDem_stShutOff>"
  sig_Result_Bus/1 -> BS_Result/1, specifyOutputs/2(sig_Result_Bus)
  BS_Result/1 -> ToWs_Result_Bus_Sig1/1  "<WESDem_stCrCtl>"
  BS_Result/2 -> ToWs_Result_Bus_Sig2/1  "<WESDem_stCfg>"
  BS_Result/3 -> ToWs_Result_Bus_Sig3/1  "<WESDem_stMode>"
  BS_Result/4 -> ToWs_Result_Bus_Sig4/1  "<WESDem_stModeChange>"
  BS_Result/5 -> ToWs_Result_Bus_Sig5/1  "<WESDem_vMaxCfg>"
  BS_Result/6 -> ToWs_Result_Bus_Sig6/1  "<WESDem_vMaxActv>"
  BS_Result/7 -> ToWs_Result_Bus_Sig7/1  "<WESDem_stShutOff>"
  specifyOutputs/1(result) -> result/1

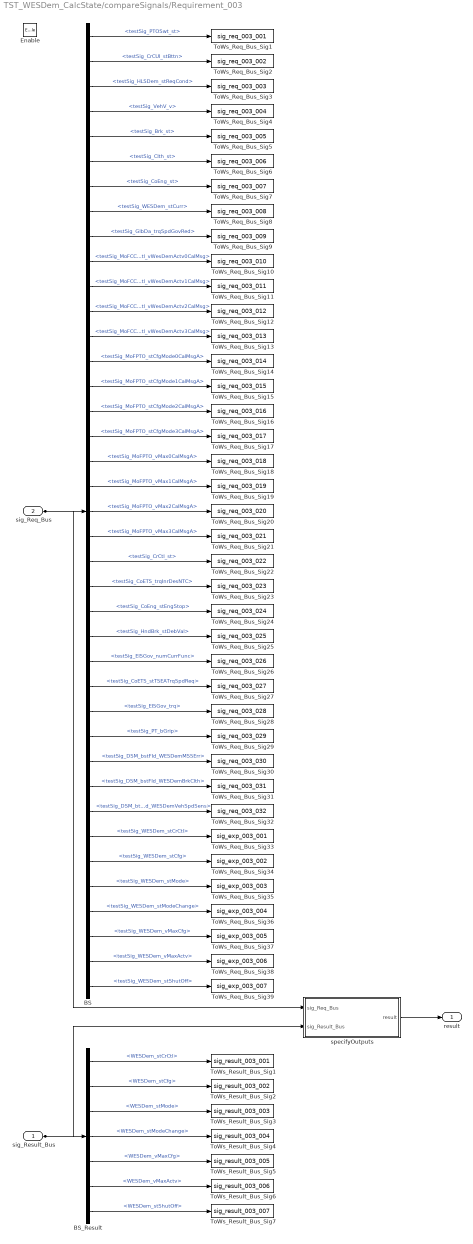
== system TST_WESDem_CalcState/compareSignals/Requirement_003 ==
  sig_Result_Bus : Inport
  sig_Req_Bus : Inport  Port=2
  Enable : EnablePort
  BS : BusSelector  OutputSignals=testSig_PTOSwt_st,testSig_CrCUI_stBttn,testSig_HLSDem_stReqCond,testSig_VehV_v,testSig_Brk_st,testSig_Clth_st,testSig_CoEng_st,testSig_WESDem_stCurr,testSig_GlbDa_trqSpdGovRed,testSig_MoFCCtl_vWesDemActv0CalMsg,testSig_MoFCCtl_vWesDemActv1CalMsg,testSig_MoFCCtl_vWesDemActv2CalMsg,testSig_MoFCCtl_vWesDemActv3CalMsg,testSig_MoFPTO_stCfgMode0CalMsgA,testSig_MoFPTO_stCfgMode1CalMsgA,testSig_MoFPTO_stCfgMode2CalMsgA,testSig_MoFPTO_stCfgMode3CalMsgA,testSig_MoFPTO_vMax0CalMsgA,testSig_MoFPTO_vMax1CalMsgA,testSig_MoFPTO_vMax2CalMsgA,testSig_MoFPTO_vMax3CalMsgA,testSig_CrCtl_st,testSig_CoETS_trqInrDesNTC,testSig_CoEng_stEngStop,testSig_HndBrk_stDebVal,testSig_EISGov_numCurrFunc,testSig_CoETS_stTSEATrqSpdReq,testSig_EISGov_trq,testSig_PT_bGrip,testSig_DSM_bstFId_WESDemMSSErr,testSig_DSM_bstFId_WESDemBrkClth,testSig_DSM_btFId_WESDemVehSpdSens,testSig_WESDem_stCrCtl,testSig_WESDem_stCfg,testSig_WESDem_stMode,testSig_WESDem_stModeChange,testSig_WESDem_vMaxCfg,testSig_WESDem_vMaxActv,testSig_WESDem_stShutOff
  BS_Result : BusSelector  OutputSignals=WESDem_stCrCtl,WESDem_stCfg,WESDem_stMode,WESDem_stModeChange,WESDem_vMaxCfg,WESDem_vMaxActv,WESDem_stShutOff
  ToWs_Req_Bus_Sig1 : ToWorkspace  VariableName=sig_req_003_001  SaveFormat=Structure With Time
  ToWs_Req_Bus_Sig10 : ToWorkspace  VariableName=sig_req_003_010  SaveFormat=Structure With Time
  ToWs_Req_Bus_Sig11 : ToWorkspace  VariableName=sig_req_003_011  SaveFormat=Structure With Time
  ToWs_Req_Bus_Sig12 : ToWorkspace  VariableName=sig_req_003_012  SaveFormat=Structure With Time
  ToWs_Req_Bus_Sig13 : ToWorkspace  VariableName=sig_req_003_013  SaveFormat=Structure With Time
  ToWs_Req_Bus_Sig14 : ToWorkspace  VariableName=sig_req_003_014  SaveFormat=Structure With Time
  ToWs_Req_Bus_Sig15 : ToWorkspace  VariableName=sig_req_003_015  SaveFormat=Structure With Time
  ToWs_Req_Bus_Sig16 : ToWorkspace  VariableName=sig_req_003_016  SaveFormat=Structure With Time
  ToWs_Req_Bus_Sig17 : ToWorkspace  VariableName=sig_req_003_017  SaveFormat=Structure With Time
  ToWs_Req_Bus_Sig18 : ToWorkspace  VariableName=sig_req_003_018  SaveFormat=Structure With Time
  ToWs_Req_Bus_Sig19 : ToWorkspace  VariableName=sig_req_003_019  SaveFormat=Structure With Time
  ToWs_Req_Bus_Sig2 : ToWorkspace  VariableName=sig_req_003_002  SaveFormat=Structure With Time
  ToWs_Req_Bus_Sig20 : ToWorkspace  VariableName=sig_req_003_020  SaveFormat=Structure With Time
  ToWs_Req_Bus_Sig21 : ToWorkspace  VariableName=sig_req_003_021  SaveFormat=Structure With Time
  ToWs_Req_Bus_Sig22 : ToWorkspace  VariableName=sig_req_003_022  SaveFormat=Structure With Time
  ToWs_Req_Bus_Sig23 : ToWorkspace  VariableName=sig_req_003_023  SaveFormat=Structure With Time
  ToWs_Req_Bus_Sig24 : ToWorkspace  VariableName=sig_req_003_024  SaveFormat=Structure With Time
  ToWs_Req_Bus_Sig25 : ToWorkspace  VariableName=sig_req_003_025  SaveFormat=Structure With Time
  ToWs_Req_Bus_Sig26 : ToWorkspace  VariableName=sig_req_003_026  SaveFormat=Structure With Time
  ToWs_Req_Bus_Sig27 : ToWorkspace  VariableName=sig_req_003_027  SaveFormat=Structure With Time
  ToWs_Req_Bus_Sig28 : ToWorkspace  VariableName=sig_req_003_028  SaveFormat=Structure With Time
  ToWs_Req_Bus_Sig29 : ToWorkspace  VariableName=sig_req_003_029  SaveFormat=Structure With Time
  ToWs_Req_Bus_Sig3 : ToWorkspace  VariableName=sig_req_003_003  SaveFormat=Structure With Time
  ToWs_Req_Bus_Sig30 : ToWorkspace  VariableName=sig_req_003_030  SaveFormat=Structure With Time
  ToWs_Req_Bus_Sig31 : ToWorkspace  VariableName=sig_req_003_031  SaveFormat=Structure With Time
  ToWs_Req_Bus_Sig32 : ToWorkspace  VariableName=sig_req_003_032  SaveFormat=Structure With Time
  ToWs_Req_Bus_Sig33 : ToWorkspace  VariableName=sig_exp_003_001  SaveFormat=Structure With Time
  ToWs_Req_Bus_Sig34 : ToWorkspace  VariableName=sig_exp_003_002  SaveFormat=Structure With Time
  ToWs_Req_Bus_Sig35 : ToWorkspace  VariableName=sig_exp_003_003  SaveFormat=Structure With Time
  ToWs_Req_Bus_Sig36 : ToWorkspace  VariableName=sig_exp_003_004  SaveFormat=Structure With Time
  ToWs_Req_Bus_Sig37 : ToWorkspace  VariableName=sig_exp_003_005  SaveFormat=Structure With Time
  ToWs_Req_Bus_Sig38 : ToWorkspace  VariableName=sig_exp_003_006  SaveFormat=Structure With Time
  ToWs_Req_Bus_Sig39 : ToWorkspace  VariableName=sig_exp_003_007  SaveFormat=Structure With Time
  ToWs_Req_Bus_Sig4 : ToWorkspace  VariableName=sig_req_003_004  SaveFormat=Structure With Time
  ToWs_Req_Bus_Sig5 : ToWorkspace  VariableName=sig_req_003_005  SaveFormat=Structure With Time
  ToWs_Req_Bus_Sig6 : ToWorkspace  VariableName=sig_req_003_006  SaveFormat=Structure With Time
  ToWs_Req_Bus_Sig7 : ToWorkspace  VariableName=sig_req_003_007  SaveFormat=Structure With Time
  ToWs_Req_Bus_Sig8 : ToWorkspace  VariableName=sig_req_003_008  SaveFormat=Structure With Time
  ToWs_Req_Bus_Sig9 : ToWorkspace  VariableName=sig_req_003_009  SaveFormat=Structure With Time
  ToWs_Result_Bus_Sig1 : ToWorkspace  VariableName=sig_result_003_001  SaveFormat=Structure With Time
  ToWs_Result_Bus_Sig2 : ToWorkspace  VariableName=sig_result_003_002  SaveFormat=Structure With Time
  ToWs_Result_Bus_Sig3 : ToWorkspace  VariableName=sig_result_003_003  SaveFormat=Structure With Time
  ToWs_Result_Bus_Sig4 : ToWorkspace  VariableName=sig_result_003_004  SaveFormat=Structure With Time
  ToWs_Result_Bus_Sig5 : ToWorkspace  VariableName=sig_result_003_005  SaveFormat=Structure With Time
  ToWs_Result_Bus_Sig6 : ToWorkspace  VariableName=sig_result_003_006  SaveFormat=Structure With Time
  ToWs_Result_Bus_Sig7 : ToWorkspace  VariableName=sig_result_003_007  SaveFormat=Structure With Time
  specifyOutputs : Subsystem
  result : Outport
  wires:
  sig_Req_Bus/1 -> BS/1, specifyOutputs/1(sig_Req_Bus)
  BS/1 -> ToWs_Req_Bus_Sig1/1  "<testSig_PTOSwt_st>"
  BS/2 -> ToWs_Req_Bus_Sig2/1  "<testSig_CrCUI_stBttn>"
  BS/3 -> ToWs_Req_Bus_Sig3/1  "<testSig_HLSDem_stReqCond>"
  BS/4 -> ToWs_Req_Bus_Sig4/1  "<testSig_VehV_v>"
  BS/5 -> ToWs_Req_Bus_Sig5/1  "<testSig_Brk_st>"
  BS/6 -> ToWs_Req_Bus_Sig6/1  "<testSig_Clth_st>"
  BS/7 -> ToWs_Req_Bus_Sig7/1  "<testSig_CoEng_st>"
  BS/8 -> ToWs_Req_Bus_Sig8/1  "<testSig_WESDem_stCurr>"
  BS/9 -> ToWs_Req_Bus_Sig9/1  "<testSig_GlbDa_trqSpdGovRed>"
  BS/10 -> ToWs_Req_Bus_Sig10/1  "<testSig_MoFCCtl_vWesDemActv0CalMsg>"
  BS/11 -> ToWs_Req_Bus_Sig11/1  "<testSig_MoFCCtl_vWesDemActv1CalMsg>"
  BS/12 -> ToWs_Req_Bus_Sig12/1  "<testSig_MoFCCtl_vWesDemActv2CalMsg>"
  BS/13 -> ToWs_Req_Bus_Sig13/1  "<testSig_MoFCCtl_vWesDemActv3CalMsg>"
  BS/14 -> ToWs_Req_Bus_Sig14/1  "<testSig_MoFPTO_stCfgMode0CalMsgA>"
  BS/15 -> ToWs_Req_Bus_Sig15/1  "<testSig_MoFPTO_stCfgMode1CalMsgA>"
  BS/16 -> ToWs_Req_Bus_Sig16/1  "<testSig_MoFPTO_stCfgMode2CalMsgA>"
  BS/17 -> ToWs_Req_Bus_Sig17/1  "<testSig_MoFPTO_stCfgMode3CalMsgA>"
  BS/18 -> ToWs_Req_Bus_Sig18/1  "<testSig_MoFPTO_vMax0CalMsgA>"
  BS/19 -> ToWs_Req_Bus_Sig19/1  "<testSig_MoFPTO_vMax1CalMsgA>"
  BS/20 -> ToWs_Req_Bus_Sig20/1  "<testSig_MoFPTO_vMax2CalMsgA>"
  BS/21 -> ToWs_Req_Bus_Sig21/1  "<testSig_MoFPTO_vMax3CalMsgA>"
  BS/22 -> ToWs_Req_Bus_Sig22/1  "<testSig_CrCtl_st>"
  BS/23 -> ToWs_Req_Bus_Sig23/1  "<testSig_CoETS_trqInrDesNTC>"
  BS/24 -> ToWs_Req_Bus_Sig24/1  "<testSig_CoEng_stEngStop>"
  BS/25 -> ToWs_Req_Bus_Sig25/1  "<testSig_HndBrk_stDebVal>"
  BS/26 -> ToWs_Req_Bus_Sig26/1  "<testSig_EISGov_numCurrFunc>"
  BS/27 -> ToWs_Req_Bus_Sig27/1  "<testSig_CoETS_stTSEATrqSpdReq>"
  BS/28 -> ToWs_Req_Bus_Sig28/1  "<testSig_EISGov_trq>"
  BS/29 -> ToWs_Req_Bus_Sig29/1  "<testSig_PT_bGrip>"
  BS/30 -> ToWs_Req_Bus_Sig30/1  "<testSig_DSM_bstFId_WESDemMSSErr>"
  BS/31 -> ToWs_Req_Bus_Sig31/1  "<testSig_DSM_bstFId_WESDemBrkClth>"
  BS/32 -> ToWs_Req_Bus_Sig32/1  "<testSig_DSM_btFId_WESDemVehSpdSens>"
  BS/33 -> ToWs_Req_Bus_Sig33/1  "<testSig_WESDem_stCrCtl>"
  BS/34 -> ToWs_Req_Bus_Sig34/1  "<testSig_WESDem_stCfg>"
  BS/35 -> ToWs_Req_Bus_Sig35/1  "<testSig_WESDem_stMode>"
  BS/36 -> ToWs_Req_Bus_Sig36/1  "<testSig_WESDem_stModeChange>"
  BS/37 -> ToWs_Req_Bus_Sig37/1  "<testSig_WESDem_vMaxCfg>"
  BS/38 -> ToWs_Req_Bus_Sig38/1  "<testSig_WESDem_vMaxActv>"
  BS/39 -> ToWs_Req_Bus_Sig39/1  "<testSig_WESDem_stShutOff>"
  sig_Result_Bus/1 -> BS_Result/1, specifyOutputs/2(sig_Result_Bus)
  BS_Result/1 -> ToWs_Result_Bus_Sig1/1  "<WESDem_stCrCtl>"
  BS_Result/2 -> ToWs_Result_Bus_Sig2/1  "<WESDem_stCfg>"
  BS_Result/3 -> ToWs_Result_Bus_Sig3/1  "<WESDem_stMode>"
  BS_Result/4 -> ToWs_Result_Bus_Sig4/1  "<WESDem_stModeChange>"
  BS_Result/5 -> ToWs_Result_Bus_Sig5/1  "<WESDem_vMaxCfg>"
  BS_Result/6 -> ToWs_Result_Bus_Sig6/1  "<WESDem_vMaxActv>"
  BS_Result/7 -> ToWs_Result_Bus_Sig7/1  "<WESDem_stShutOff>"
  specifyOutputs/1(result) -> result/1
